simulink model "homework5_2"  (R2023a)
settings: Solver=VariableStepAuto  StartTime=0.0  StopTime=3  RelTol=1e-3
libraries: spsSeriesRLCBranchLib x2, spsVoltageMeasurementLib x2, spsDCVoltageSourceLib x1, spsDiodeLib x1, spsGroundLib x1, spsIGBTLib x1, spsLinearTransformerLib x1, spsMultimeterLib x1, eePwmGenerator x1, sps_lib x1
settings Model: Creator=zou20  LastModifiedBy=zou20

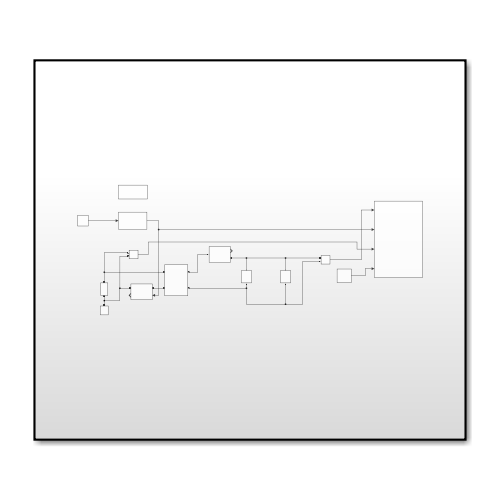
[thumbnail: Simulink's stored preview of the top-level diagram]
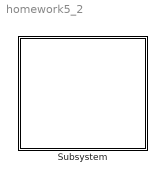
== system homework5_2 ==
  Subsystem : Subsystem

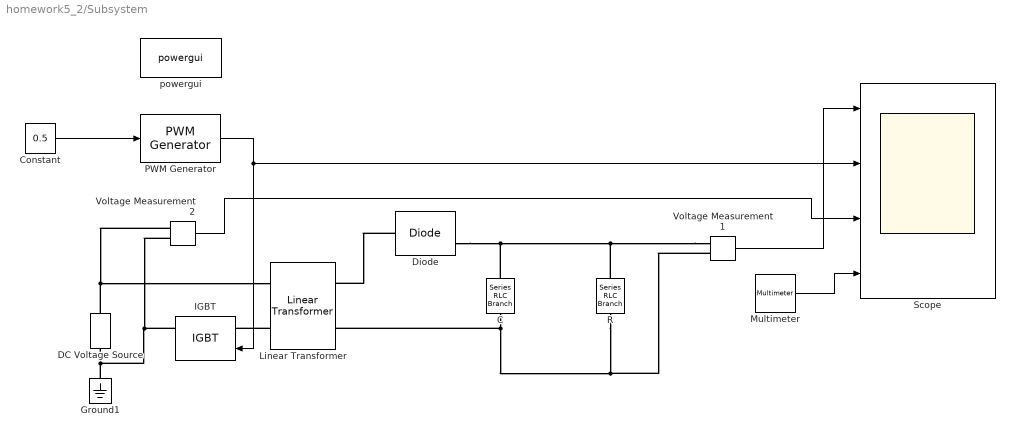
== system homework5_2/Subsystem ==
  C : spsSeriesRLCBranchLib/Series RLC Branch  LConnTagsString=__new0  RConnTagsString=__new0  BranchType=C  Resistance=0  Inductance=0  SetiL0=off  InitialCurrent=0  Capacitance=30e-4  Setx0=off  InitialVoltage=0  Measurements=Branch voltage and current
  Constant : Constant  Value=0.5
  DC Voltage Source : spsDCVoltageSourceLib/DC Voltage Source  Amplitude=200  Measurements=None
  Diode : spsDiodeLib/Diode  Ron=0.001  Lon=0  Vf=0.8  IC=0  UseSnubber=0  Rs=500  Cs=250e-9  Measurements=on
  Ground1 : spsGroundLib/Ground  LConnTagsString=a
  IGBT : spsIGBTLib/IGBT  Ron=0.001  Lon=0  Vf=1  Tf=1e-6  Tt=2e-6  IC=0  Rs=1e5  Cs=inf  Measurements=on
  Linear Transformer : spsLinearTransformerLib/Linear Transformer  UNITS=pu  NominalPower=[ 250e6 60 ]  winding1="[ 315e3  0  0 ]"  winding2="[ 315e3  0  0 ]"  ThreeWindings=off  winding3=[ 315e3 0.002 0.08 ]  RmLm=[ 500 500 ]  Measurements=All voltages and currents  DataType=off
  Multimeter : spsMultimeterLib/Multimeter  L=11  sel=[7 8]  yselected={}  Gain=[1 1]  OutputType=Complex  PlotAtSimulationStop=off  PhasorSimulation=off
  PWM Generator : eePwmGenerator/PWM Generator  CarrCount=Up  Tper=0.05  Tdelay=0  Ts=5e-5
  R : spsSeriesRLCBranchLib/Series RLC Branch  LConnTagsString=__new0  RConnTagsString=__new0  BranchType=R  Resistance=40  Inductance=0  SetiL0=off  InitialCurrent=0  Capacitance=0  Setx0=off  InitialVoltage=0  Measurements=Branch voltage and current
  Scope : Scope  NumInputPorts=4
  Voltage Measurement1 : spsVoltageMeasurementLib/Voltage Measurement  PhasorSimulation=off  OutputType=Complex  PSBequivalent=0
  Voltage Measurement2 : spsVoltageMeasurementLib/Voltage Measurement  PhasorSimulation=off  OutputType=Complex  PSBequivalent=0
  powergui : sps_lib/powergui  Priority=1  SimulationMode=Continuous  SampleTime=50e-6  frequency=60  Iterations=50  frequencyindice=0  Pbase=100e6  ErrMax=1e-4  UnitsV=kV  UnitsW=MW  buscounter=0  FunctionMessages=off  echomessages=off  EnableUseOfTLC=off  CurrentSourceSwitches=off  DisableSnubberDevices=off  DisableRonSwitches=off  DisableVfSwitches=off  DisplayEquations=off  AutomaticDiscreteSolvers=off  SolverType=Tustin/Backward Euler (TBE)  Interpol=off  ExternalGateDelay=off  methode=off  Ts=100  x0status=blocks  SPID=on  SwTol=0  HookPort=off  NonlinearTolerance=1e-4  nMaxIteration=100  ContinueOnMaxIteration=off  RestoreLinks=warning  ResistiveCurrentMeasurement=off  Frange=[0:2:500]  Ylog=off  Xlog=on  ShowGrid=off  save=off  variable=ZData  structure=0  ZoomFFT=off  StartTime=0.0  cycles=1  DisplayStyle=1  fundamental=60  FreqAxis=off  MaxFrequency=1000  frequencyindicesteady=1  RmsSteady=1  display=off
  wires:
  Constant/1 -> PWM Generator/1
  Voltage Measurement1/1 -> Scope/1
  PWM Generator/1 -> IGBT/1, Scope/2
  Voltage Measurement2/1 -> Scope/3
  Multimeter/1 -> Scope/4
  connections:
  Voltage Measurement1/LConn1 -- R/RConn1 -- Diode/RConn1 -- C/RConn1
  DC Voltage Source/RConn1 -- Voltage Measurement2/LConn1 -- Linear Transformer/LConn1
  Voltage Measurement1/LConn2 -- R/LConn1 -- C/LConn1 -- Linear Transformer/RConn2
  Linear Transformer/LConn2 -- IGBT/LConn1
  IGBT/RConn1 -- Voltage Measurement2/LConn2 -- Ground1/LConn1 -- DC Voltage Source/LConn1
  Diode/LConn1 -- Linear Transformer/RConn1
